simulink library "flightGearInterfaceLibrary"  (R2024a)
settings: Solver=VariableStepAuto  StartTime=0.0  StopTime=10.0  RelTol=1e-3
settings Model: Creator=jerem  LastModifiedBy=jerem

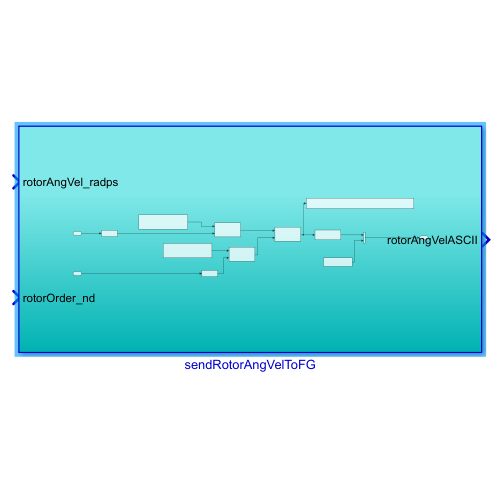
[thumbnail: Simulink's stored preview of the top-level diagram]
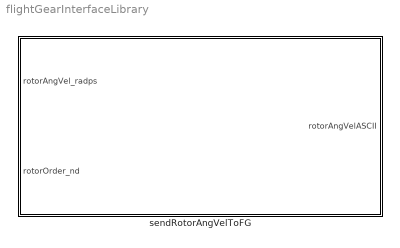
== system flightGearInterfaceLibrary ==
  sendRotorAngVelToFG : Subsystem

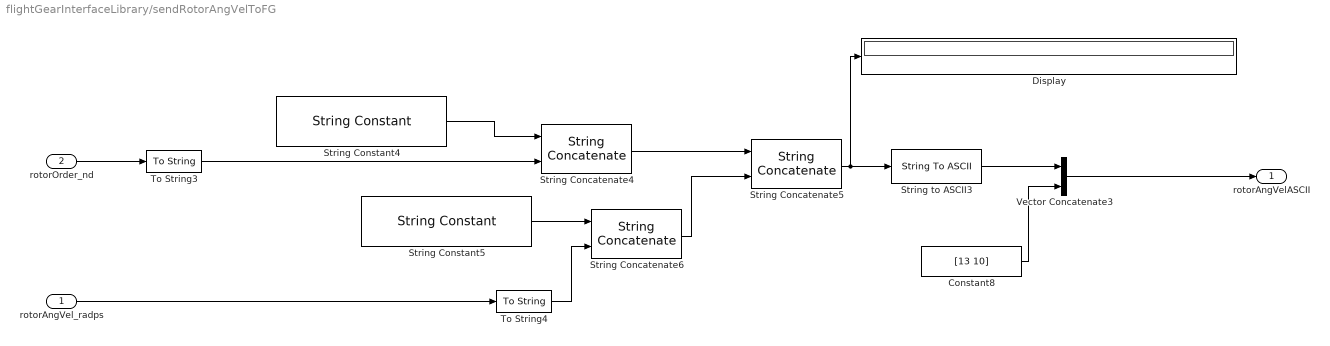
== system flightGearInterfaceLibrary/sendRotorAngVelToFG ==
  rotorAngVel_radps : Inport
  rotorOrder_nd : Inport  Port=2
  Constant8 : Constant  Value=[13 10]  OutDataTypeStr=uint8
  Display : Display
  String Concatenate4 : StringConcatenate
  String Concatenate5 : StringConcatenate
  String Concatenate6 : StringConcatenate
  String Constant4 : StringConstant  String="\"set /engines/engine[\""
  String Constant5 : StringConstant  String="\"]/rpm \""
  String to ASCII3 : StringToASCII  OutputVectorSize=30
  To String3 : ToString
  To String4 : ToString
  Vector Concatenate3 : Concatenate
  rotorAngVelASCII : Outport
  wires:
  String to ASCII3/1 -> Vector Concatenate3/1
  To String4/1 -> String Concatenate6/2
  Constant8/1 -> Vector Concatenate3/2
  String Concatenate6/1 -> String Concatenate5/2
  String Constant4/1 -> String Concatenate4/1
  String Concatenate5/1 -> Display/1, String to ASCII3/1
  String Concatenate4/1 -> String Concatenate5/1
  String Constant5/1 -> String Concatenate6/1
  To String3/1 -> String Concatenate4/2
  Vector Concatenate3/1 -> rotorAngVelASCII/1
  rotorAngVel_radps/1 -> To String4/1
  rotorOrder_nd/1 -> To String3/1
